simulink model "first"  (R2020b)
settings: Solver=VariableStepAuto  StartTime=0.0  StopTime=10.0  RelTol=1e-3
settings Model: Creator=priyaD  LastModifiedBy=priyaD

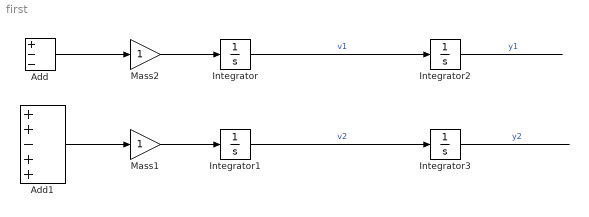
== system first ==
  Add : Sum  Inputs=+--
  Add1 : Sum  Inputs=++-++
  Integrator{,1..3} (4 alike) : Integrator
  Mass1 : Gain
  Mass2 : Gain
  wires:
  Integrator2/1 -> ?  "y1"
  Integrator3/1 -> ?  "y2"
  Integrator/1 -> Integrator2/1  "v1"
  Integrator1/1 -> Integrator3/1  "v2"
  Mass2/1 -> Integrator/1
  Mass1/1 -> Integrator1/1
  Add/1 -> Mass2/1
  Add1/1 -> Mass1/1
